simulink model "MIL4L3_SW6_V1_20220211"  (R2018b)
settings: Solver=FixedStepAuto  StartTime=0.0  StopTime=inf  FixedStep=0.001  RelTol=1e-3
PreLoadFcn:
  | A0_MILtest;
undefined symbols (not defined in the file or in its folder): Clb_ICADirect_LaneDisp_StateFive, Clb_ICADirect_LaneDisp_StateFour, Clb_ICADirect_LaneDisp_StateOne, Clb_ICADirect_LaneDisp_StateThree, Clb_ICADirect_LaneDisp_StateTwo, Clb_ICADirect_LaneDisp_StateZero, Clb_ICADirect_LaneDispSW, Clb_ICADirect_TrnLghtsCom_Switch, Clb_ICADirect_TrnLghtsCom_Value, Clb_ICADirect_TrnLghtsCrtl_Inhb, IMAP_Clb_ACU_Driver_Belt, IMAP_Clb_ACU_Driver_Belt_Over, IMAP_Clb_ACU_Passenger_Belt, IMAP_Clb_ACU_Passenger_Belt_Over, IMAP_Clb_ACU_RearLeft_Belt, IMAP_Clb_ACU_RearLeft_Belt_Over, IMAP_Clb_ACU_RearMiddle_Belt, IMAP_Clb_ACU_RearMiddle_Belt_Over, IMAP_Clb_ACU_RearRight_Belt, IMAP_Clb_ACU_RearRight_Belt_Over, IMAP_Clb_AEB_Switch, IMAP_Clb_AEB_Switch_Over, IMAP_Clb_ALC_TLC_Mode, IMAP_Clb_ALC_TLC_Mode_Over, IMAP_Clb_BCM_Battery_Voltage, IMAP_Clb_BCM_Battery_Voltage_Over, IMAP_Clb_BCM_BrakeLamp_State, IMAP_Clb_BCM_BrakeLamp_State_Over, IMAP_Clb_BCM_CHMSL_Status, IMAP_Clb_BCM_CHMSL_Status_Over, IMAP_Clb_BCM_Door_Lock_State, IMAP_Clb_BCM_Door_Lock_State_Over, IMAP_Clb_BCM_FrontWiper_State, IMAP_Clb_BCM_FrontWiper_State_Over, IMAP_Clb_BCM_FrontWiper_Switch, IMAP_Clb_BCM_FrontWiper_Switch_Over, IMAP_Clb_BCM_HazardLamp, IMAP_Clb_BCM_HazardLamp_Over, IMAP_Clb_BCM_HazardLamp_Switch, IMAP_Clb_BCM_HazardLamp_Switch_Over, IMAP_Clb_BCM_HighBeam_State, IMAP_Clb_BCM_HighBeam_State_Over, IMAP_Clb_BCM_Ignition_State, IMAP_Clb_BCM_Ignition_State_Over, IMAP_Clb_BCM_IHBC_Enabled, IMAP_Clb_BCM_IHBC_Enabled_Over, IMAP_Clb_BCM_Left_Light, IMAP_Clb_BCM_Left_Light_Over, IMAP_Clb_BCM_LeftTurn_Switch, IMAP_Clb_BCM_LeftTurn_Switch_Over, IMAP_Clb_BCM_LF_Door_State, IMAP_Clb_BCM_LF_Door_State_Over, IMAP_Clb_BCM_LowBeam_State, IMAP_Clb_BCM_LowBeam_State_Over, IMAP_Clb_BCM_LR_Door_State, IMAP_Clb_BCM_LR_Door_State_Over, IMAP_Clb_BCM_RF_Door_State, IMAP_Clb_BCM_RF_Door_State_Over, IMAP_Clb_BCM_Right_Light, IMAP_Clb_BCM_Right_Light_Over ... (+547)
libraries: CarMaker4SL x2153, simulink x292, dspstat3 x3, canmsglib x2, simulink_extras x1
(part 51 of 52)

== system MIL4L3_SW6_V1_20220211/CarMaker/VehicleControl/Function/LKA/LKAS1/LL/LLOn/LL State Determination (LLStateDet)/LL State Machine Conditions (LLSMCon)/Deactivation Condition (DeactvC)/Deviation Threshold Condition (DvtThresCon)/Deviation Threshold Judgement LKA (DvtThresJdg)/Deviation Speed Detection (DvtSpdDet)/Ph2SWA ==
  Action Port : ActionPort  InitializeStates=reset  ActionType=elseif
      settings: AttributesFormatString=states = %<InitializeStates>
  Constant : Constant  Value=-1  OutDataTypeStr=single
  Out : Outport
      settings: AttributesFormatString=%<OutputWhenDisabled> = %<InitialOutput>
  wires:
  Constant/1 -> Out/1

== system MIL4L3_SW6_V1_20220211/CarMaker/VehicleControl/Function/LKA/LKAS1/LL/LLOn/LL State Determination (LLStateDet)/LL State Machine Conditions (LLSMCon)/Deactivation Condition (DeactvC)/Deviation Threshold Condition (DvtThresCon)/Deviation Threshold Judgement LKA (DvtThresJdg)/Deviation Speed Detection (DvtSpdDet)/Ph3SWA ==
  Action Port : ActionPort  InitializeStates=reset  ActionType=else
      settings: AttributesFormatString=states = %<InitializeStates>
  Constant : Constant  Value=0  OutDataTypeStr=single
  Out : Outport
      settings: AttributesFormatString=%<OutputWhenDisabled> = %<InitialOutput>
  wires:
  Constant/1 -> Out/1

== system MIL4L3_SW6_V1_20220211/CarMaker/VehicleControl/Function/LKA/LKAS1/LL/LLOn/LL State Determination (LLStateDet)/LL State Machine Conditions (LLSMCon)/Disable Condition (DisblC)/Driver Intent Condition (DrvInttC)/Take-Over Steering Check (TkOvStChk)/Time Delay (TDel)/If Action Subsystem ==
  Action Port : ActionPort  InitializeStates=reset  ActionType=then
      settings: AttributesFormatString=states = %<InitializeStates>
  Constant : Constant  OutDataTypeStr=boolean  SampleTime=-1
  Out : Outport
      settings: AttributesFormatString=%<OutputWhenDisabled> = %<InitialOutput>
  wires:
  Constant/1 -> Out/1

== system MIL4L3_SW6_V1_20220211/CarMaker/VehicleControl/Function/LKA/LKAS1/LL/LLOn/LL State Determination (LLStateDet)/LL State Machine Conditions (LLSMCon)/Disable Condition (DisblC)/Driver Intent Condition (DrvInttC)/Take-Over Steering Check (TkOvStChk)/Time Delay (TDel)/If Action Subsystem3 ==
  In1 : Inport
  Action Port : ActionPort  InitializeStates=reset  ActionType=else
      settings: AttributesFormatString=states = %<InitializeStates>
  Out : Outport
      settings: AttributesFormatString=%<OutputWhenDisabled> = %<InitialOutput>
  wires:
  In1/1 -> Out/1

== system MIL4L3_SW6_V1_20220211/CarMaker/VehicleControl/Function/LKA/LKAS1/LL/LLOn/LL State Determination (LLStateDet)/LL State Machine Conditions (LLSMCon)/Disable Condition (DisblC)/Driver Intent Condition (DrvInttC)/Take-Over Steering Check (TkOvStChk)/Time Delay (TDel)/Sum Condition1 ==
  SampleTime : Inport
  Sum : Inport  Port=2
  state = reset : EnablePort  StatesWhenEnabling=reset
  Add1 : Sum  OutDataTypeStr=single
  Memory : Memory  InheritSampleTime=on
  Relational Operator : RelationalOperator  Operator=<=  OutDataTypeStr=boolean  RndMeth=Nearest
  Saturation : Saturate  UpperLimit=10  LowerLimit=0
      settings: AttributesFormatString="Min = %<LowerLimit>  Max = %<UpperLimit>"
  Out : Outport  OutputWhenDisabled=reset  InitialOutput=0
      settings: AttributesFormatString=%<OutputWhenDisabled> = %<InitialOutput>
  wires:
  Memory/1 -> Add1/2
  Add1/1 -> Saturation/1
  SampleTime/1 -> Add1/1
  Sum/1 -> Relational Operator/2
  Relational Operator/1 -> Out/1
  Saturation/1 -> Memory/1, Relational Operator/1

== system MIL4L3_SW6_V1_20220211/CarMaker/VehicleControl/OMAP/OMAP1/Runnable_OMAP_10ms_sys/OMAP_Module/ICA_Direct_G59/ICA_Define/Subsystem1/Dspl/DsplPrcs/Txt/TxtActv/Hold ==
  In1 : Inport
  Action Port : ActionPort  ActionType=else
  Out1 : Outport
  wires:
  In1/1 -> Out1/1

== system MIL4L3_SW6_V1_20220211/CarMaker/VehicleControl/OMAP/OMAP1/Runnable_OMAP_10ms_sys/OMAP_Module/ICA_Direct_G59/ICA_Define/Subsystem1/Dspl/DsplPrcs/Txt/TxtActv/Start ==
  In1 : Inport
  Action Port : ActionPort  ActionType=then
  Out1 : Outport
  wires:
  In1/1 -> Out1/1

== system MIL4L3_SW6_V1_20220211/CarMaker/VehicleControl/OMAP/OMAP1/Runnable_OMAP_10ms_sys/OMAP_Module/ICA_Direct_G59/ICA_Define/Subsystem1/Dspl/DsplPrcs/Txt/TxtActv/Stop ==
  In1 : Inport
  Action Port : ActionPort  ActionType=elseif
  Out1 : Outport
  wires:
  In1/1 -> Out1/1

== system MIL4L3_SW6_V1_20220211/CarMaker/VehicleControl/OMAP/OMAP1/Runnable_OMAP_10ms_sys/OMAP_Module/ICA_Direct_G59/ICA_Define/Subsystem1/Dspl/DsplPrcs/Txt/TxtCncl/Hold ==
  In1 : Inport
  Action Port : ActionPort  ActionType=else
  Out1 : Outport
  wires:
  In1/1 -> Out1/1

== system MIL4L3_SW6_V1_20220211/CarMaker/VehicleControl/OMAP/OMAP1/Runnable_OMAP_10ms_sys/OMAP_Module/ICA_Direct_G59/ICA_Define/Subsystem1/Dspl/DsplPrcs/Txt/TxtCncl/Start ==
  In1 : Inport
  Action Port : ActionPort  ActionType=then
  Out1 : Outport
  wires:
  In1/1 -> Out1/1

== system MIL4L3_SW6_V1_20220211/CarMaker/VehicleControl/OMAP/OMAP1/Runnable_OMAP_10ms_sys/OMAP_Module/ICA_Direct_G59/ICA_Define/Subsystem1/Dspl/DsplPrcs/Txt/TxtCncl/Stop ==
  In1 : Inport
  Action Port : ActionPort  ActionType=elseif
  Out1 : Outport
  wires:
  In1/1 -> Out1/1

== system MIL4L3_SW6_V1_20220211/CarMaker/VehicleControl/OMAP/OMAP1/Runnable_OMAP_10ms_sys/OMAP_Module/ICA_Direct_G59/ICA_Define/Subsystem1/Dspl/DsplPrcs/Txt/TxtDegraded/Hold ==
  In1 : Inport
  Action Port : ActionPort  ActionType=else
  Out1 : Outport
  wires:
  In1/1 -> Out1/1

== system MIL4L3_SW6_V1_20220211/CarMaker/VehicleControl/OMAP/OMAP1/Runnable_OMAP_10ms_sys/OMAP_Module/ICA_Direct_G59/ICA_Define/Subsystem1/Dspl/DsplPrcs/Txt/TxtDegraded/Start ==
  In1 : Inport
  Action Port : ActionPort  ActionType=then
  Out1 : Outport
  wires:
  In1/1 -> Out1/1

== system MIL4L3_SW6_V1_20220211/CarMaker/VehicleControl/OMAP/OMAP1/Runnable_OMAP_10ms_sys/OMAP_Module/ICA_Direct_G59/ICA_Define/Subsystem1/Dspl/DsplPrcs/Txt/TxtDegraded/Stop ==
  In1 : Inport
  Action Port : ActionPort  ActionType=elseif
  Out1 : Outport
  wires:
  In1/1 -> Out1/1

== system MIL4L3_SW6_V1_20220211/CarMaker/VehicleControl/OMAP/OMAP1/Runnable_OMAP_10ms_sys/OMAP_Module/ICA_Direct_G59/ICA_Define/Subsystem1/Dspl/DsplPrcs/Txt/TxtFromACC/Enabled Subsystem ==
  Num : Inport
  Enable : EnablePort  StatesWhenEnabling=reset
  Add : Sum
  Constant : Constant  OutDataTypeStr=single
  Constant1 : Constant  Value=0  OutDataTypeStr=single
  Delay : Delay  DelayLength=1  InitialCondition=0
  Gain : Gain  Gain=2  ParamDataTypeStr=single
  Relational Operator : RelationalOperator  Operator=<=  OutDataTypeStr=boolean  RndMeth=Nearest
  Saturation Dynamic : simulink/Discontinuities/Saturation Dynamic  OutMin=[]  OutMax=[]  OutDataTypeStr=Inherit: Same as second input  OutDataType=fixdt(1, 16)  OutScaling=2^-10  DoSatur=off
  Triger : Outport  OutputWhenDisabled=reset  InitialOutput=single(0)
  wires:
  Constant/1 -> Add/1
  Delay/1 -> Add/2
  Add/1 -> Saturation Dynamic/2
  Saturation Dynamic/1 -> Relational Operator/2, Delay/1
  Constant1/1 -> Saturation Dynamic/3
  Num/1 -> Relational Operator/1, Gain/1
  Gain/1 -> Saturation Dynamic/1
  Relational Operator/1 -> Triger/1

== system MIL4L3_SW6_V1_20220211/CarMaker/VehicleControl/OMAP/OMAP1/Runnable_OMAP_10ms_sys/OMAP_Module/ICA_Direct_G59/ICA_Define/Subsystem1/Dspl/DsplPrcs/Txt/TxtFromACC/Hold ==
  In1 : Inport
  Action Port : ActionPort  ActionType=else
  Out1 : Outport
  wires:
  In1/1 -> Out1/1

== system MIL4L3_SW6_V1_20220211/CarMaker/VehicleControl/OMAP/OMAP1/Runnable_OMAP_10ms_sys/OMAP_Module/ICA_Direct_G59/ICA_Define/Subsystem1/Dspl/DsplPrcs/Txt/TxtFromACC/RdrBlkInhib ==
  RdrBlkInhib_stTHState : Inport
  RdrBlkInhib_stLstTHState : Inport  Port=2
  RdrBlkInhib_stACCTxtDspl : Inport  Port=3
  Constant1 : Constant  OutDataTypeStr=uint16
  Constant2 : Constant  Value=0  OutDataTypeStr=uint16
  If : If  NumInputs=3  IfExpression=u1 == 5 & u2 == 0 & u3 == 2  ElseIfExpressions=u1 ~= 5 | u3 ~= 2
  Inhibit : Subsystem  TreatAsAtomicUnit=on
  Merge : Merge  Inputs=3
  Unit Delay1 : UnitDelay  SampleTime=-1
  hold_last : Subsystem  TreatAsAtomicUnit=on
  not_Inhibit : Subsystem  TreatAsAtomicUnit=on
  RdrBlkInhib_stRdrBlkInhibFlg : Outport
  wires:
  RdrBlkInhib_stTHState/1 -> If/1
  Merge/1 -> Unit Delay1/1, RdrBlkInhib_stRdrBlkInhibFlg/1
  Inhibit/1(Out1) -> Merge/1
  RdrBlkInhib_stLstTHState/1 -> If/2
  RdrBlkInhib_stACCTxtDspl/1 -> If/3
  Constant1/1 -> Inhibit/1(In1)
  If/1 -> Inhibit/Action
  Constant2/1 -> not_Inhibit/1(In1)
  If/2 -> not_Inhibit/Action
  Unit Delay1/1 -> hold_last/1(In1)
  If/3 -> hold_last/Action
  not_Inhibit/1(Out1) -> Merge/2
  hold_last/1(Out1) -> Merge/3

== system MIL4L3_SW6_V1_20220211/CarMaker/VehicleControl/OMAP/OMAP1/Runnable_OMAP_10ms_sys/OMAP_Module/ICA_Direct_G59/ICA_Define/Subsystem1/Dspl/DsplPrcs/Txt/TxtFromACC/Start ==
  In1 : Inport
  Action Port : ActionPort  ActionType=then
  Out1 : Outport
  wires:
  In1/1 -> Out1/1

== system MIL4L3_SW6_V1_20220211/CarMaker/VehicleControl/OMAP/OMAP1/Runnable_OMAP_10ms_sys/OMAP_Module/ICA_Direct_G59/ICA_Define/Subsystem1/Dspl/DsplPrcs/Txt/TxtFromACC/Start1 ==
  In1 : Inport
  Action Port : ActionPort  ActionType=then
  Out1 : Outport
  wires:
  In1/1 -> Out1/1

== system MIL4L3_SW6_V1_20220211/CarMaker/VehicleControl/OMAP/OMAP1/Runnable_OMAP_10ms_sys/OMAP_Module/ICA_Direct_G59/ICA_Define/Subsystem1/Dspl/DsplPrcs/Txt/TxtFromACC/Start2 ==
  In1 : Inport
  Action Port : ActionPort  ActionType=then
  Out1 : Outport
  wires:
  In1/1 -> Out1/1

== system MIL4L3_SW6_V1_20220211/CarMaker/VehicleControl/OMAP/OMAP1/Runnable_OMAP_10ms_sys/OMAP_Module/ICA_Direct_G59/ICA_Define/Subsystem1/Dspl/DsplPrcs/Txt/TxtFromACC/Start3 ==
  In1 : Inport
  Action Port : ActionPort  ActionType=then
  Out1 : Outport
  wires:
  In1/1 -> Out1/1

== system MIL4L3_SW6_V1_20220211/CarMaker/VehicleControl/OMAP/OMAP1/Runnable_OMAP_10ms_sys/OMAP_Module/ICA_Direct_G59/ICA_Define/Subsystem1/Dspl/DsplPrcs/Txt/TxtFromACC/Start4 ==
  In1 : Inport
  Action Port : ActionPort  ActionType=then
  Out1 : Outport
  wires:
  In1/1 -> Out1/1

== system MIL4L3_SW6_V1_20220211/CarMaker/VehicleControl/OMAP/OMAP1/Runnable_OMAP_10ms_sys/OMAP_Module/ICA_Direct_G59/ICA_Define/Subsystem1/Dspl/DsplPrcs/Txt/TxtFromACC/Start5 ==
  In1 : Inport
  Action Port : ActionPort  ActionType=then
  Out1 : Outport
  wires:
  In1/1 -> Out1/1

== system MIL4L3_SW6_V1_20220211/CarMaker/VehicleControl/OMAP/OMAP1/Runnable_OMAP_10ms_sys/OMAP_Module/ICA_Direct_G59/ICA_Define/Subsystem1/Dspl/DsplPrcs/Txt/TxtFromACC/Start6 ==
  In1 : Inport
  Action Port : ActionPort  ActionType=then
  Out1 : Outport
  wires:
  In1/1 -> Out1/1

== system MIL4L3_SW6_V1_20220211/CarMaker/VehicleControl/OMAP/OMAP1/Runnable_OMAP_10ms_sys/OMAP_Module/ICA_Direct_G59/ICA_Define/Subsystem1/Dspl/DsplPrcs/Txt/TxtFromACC/Start7 ==
  In1 : Inport
  Action Port : ActionPort  ActionType=then
  Out1 : Outport
  wires:
  In1/1 -> Out1/1

== system MIL4L3_SW6_V1_20220211/CarMaker/VehicleControl/OMAP/OMAP1/Runnable_OMAP_10ms_sys/OMAP_Module/ICA_Direct_G59/ICA_Define/Subsystem1/Dspl/DsplPrcs/Txt/TxtFromACC/Start8 ==
  In1 : Inport
  Action Port : ActionPort  ActionType=then
  Out1 : Outport
  wires:
  In1/1 -> Out1/1

== system MIL4L3_SW6_V1_20220211/CarMaker/VehicleControl/OMAP/OMAP1/Runnable_OMAP_10ms_sys/OMAP_Module/ICA_Direct_G59/ICA_Define/Subsystem1/Dspl/DsplPrcs/Txt/TxtFromACC/Start9 ==
  In1 : Inport
  Action Port : ActionPort  ActionType=then
  Out1 : Outport
  wires:
  In1/1 -> Out1/1

== system MIL4L3_SW6_V1_20220211/CarMaker/VehicleControl/OMAP/OMAP1/Runnable_OMAP_10ms_sys/OMAP_Module/ICA_Direct_G59/ICA_Define/Subsystem1/Dspl/DsplPrcs/Txt/TxtFromACC/Stop ==
  In1 : Inport
  Action Port : ActionPort  ActionType=else
  Out1 : Outport
  wires:
  In1/1 -> Out1/1

== system MIL4L3_SW6_V1_20220211/CarMaker/VehicleControl/OMAP/OMAP1/Runnable_OMAP_10ms_sys/OMAP_Module/ICA_Direct_G59/ICA_Define/Subsystem1/Dspl/DsplPrcs/Txt/TxtFromACC/Stop1 ==
  In1 : Inport
  Action Port : ActionPort  ActionType=else
  Out1 : Outport
  wires:
  In1/1 -> Out1/1

== system MIL4L3_SW6_V1_20220211/CarMaker/VehicleControl/OMAP/OMAP1/Runnable_OMAP_10ms_sys/OMAP_Module/ICA_Direct_G59/ICA_Define/Subsystem1/Dspl/DsplPrcs/Txt/TxtFromACC/Stop2 ==
  In1 : Inport
  Action Port : ActionPort  ActionType=else
  Out1 : Outport
  wires:
  In1/1 -> Out1/1

== system MIL4L3_SW6_V1_20220211/CarMaker/VehicleControl/OMAP/OMAP1/Runnable_OMAP_10ms_sys/OMAP_Module/ICA_Direct_G59/ICA_Define/Subsystem1/Dspl/DsplPrcs/Txt/TxtFromACC/Stop3 ==
  In1 : Inport
  Action Port : ActionPort  ActionType=else
  Out1 : Outport
  wires:
  In1/1 -> Out1/1

== system MIL4L3_SW6_V1_20220211/CarMaker/VehicleControl/OMAP/OMAP1/Runnable_OMAP_10ms_sys/OMAP_Module/ICA_Direct_G59/ICA_Define/Subsystem1/Dspl/DsplPrcs/Txt/TxtFromACC/Stop4 ==
  In1 : Inport
  Action Port : ActionPort  ActionType=elseif
  Out1 : Outport
  wires:
  In1/1 -> Out1/1

== system MIL4L3_SW6_V1_20220211/CarMaker/VehicleControl/OMAP/OMAP1/Runnable_OMAP_10ms_sys/OMAP_Module/ICA_Direct_G59/ICA_Define/Subsystem1/Dspl/DsplPrcs/Txt/TxtFromACC/Stop5 ==
  In1 : Inport
  Action Port : ActionPort  ActionType=else
  Out1 : Outport
  wires:
  In1/1 -> Out1/1

== system MIL4L3_SW6_V1_20220211/CarMaker/VehicleControl/OMAP/OMAP1/Runnable_OMAP_10ms_sys/OMAP_Module/ICA_Direct_G59/ICA_Define/Subsystem1/Dspl/DsplPrcs/Txt/TxtFromACC/Stop6 ==
  In1 : Inport
  Action Port : ActionPort  ActionType=else
  Out1 : Outport
  wires:
  In1/1 -> Out1/1

== system MIL4L3_SW6_V1_20220211/CarMaker/VehicleControl/OMAP/OMAP1/Runnable_OMAP_10ms_sys/OMAP_Module/ICA_Direct_G59/ICA_Define/Subsystem1/Dspl/DsplPrcs/Txt/TxtFromACC/Stop7 ==
  In1 : Inport
  Action Port : ActionPort  ActionType=else
  Out1 : Outport
  wires:
  In1/1 -> Out1/1

== system MIL4L3_SW6_V1_20220211/CarMaker/VehicleControl/OMAP/OMAP1/Runnable_OMAP_10ms_sys/OMAP_Module/ICA_Direct_G59/ICA_Define/Subsystem1/Dspl/DsplPrcs/Txt/TxtFromACC/Stop8 ==
  In1 : Inport
  Action Port : ActionPort  ActionType=else
  Out1 : Outport
  wires:
  In1/1 -> Out1/1

== system MIL4L3_SW6_V1_20220211/CarMaker/VehicleControl/OMAP/OMAP1/Runnable_OMAP_10ms_sys/OMAP_Module/ICA_Direct_G59/ICA_Define/Subsystem1/Dspl/DsplPrcs/Txt/TxtFromACC/Stop9 ==
  In1 : Inport
  Action Port : ActionPort  ActionType=else
  Out1 : Outport
  wires:
  In1/1 -> Out1/1

== system MIL4L3_SW6_V1_20220211/CarMaker/VehicleControl/OMAP/OMAP1/Runnable_OMAP_10ms_sys/OMAP_Module/ICA_Direct_G59/ICA_Define/Subsystem1/Dspl/DsplPrcs/Txt/TxtInactv/Hold ==
  In1 : Inport
  Action Port : ActionPort  ActionType=else
  Out1 : Outport
  wires:
  In1/1 -> Out1/1

== system MIL4L3_SW6_V1_20220211/CarMaker/VehicleControl/OMAP/OMAP1/Runnable_OMAP_10ms_sys/OMAP_Module/ICA_Direct_G59/ICA_Define/Subsystem1/Dspl/DsplPrcs/Txt/TxtInactv/Start ==
  In1 : Inport
  Action Port : ActionPort  ActionType=elseif
  Out1 : Outport
  wires:
  In1/1 -> Out1/1

== system MIL4L3_SW6_V1_20220211/CarMaker/VehicleControl/OMAP/OMAP1/Runnable_OMAP_10ms_sys/OMAP_Module/ICA_Direct_G59/ICA_Define/Subsystem1/Dspl/DsplPrcs/Txt/TxtInactv/Stop ==
  In1 : Inport
  Action Port : ActionPort  ActionType=then
  Out1 : Outport
  wires:
  In1/1 -> Out1/1

== system MIL4L3_SW6_V1_20220211/CarMaker/VehicleControl/OMAP/OMAP1/Runnable_OMAP_10ms_sys/OMAP_Module/ICA_Direct_G59/ICA_Define/Subsystem1/Dspl/DsplPrcs/Txt/TxtOff/Hold ==
  In1 : Inport
  Action Port : ActionPort  ActionType=else
  Out1 : Outport
  wires:
  In1/1 -> Out1/1

== system MIL4L3_SW6_V1_20220211/CarMaker/VehicleControl/OMAP/OMAP1/Runnable_OMAP_10ms_sys/OMAP_Module/ICA_Direct_G59/ICA_Define/Subsystem1/Dspl/DsplPrcs/Txt/TxtOff/Start ==
  In1 : Inport
  Action Port : ActionPort  ActionType=then
  Out1 : Outport
  wires:
  In1/1 -> Out1/1

== system MIL4L3_SW6_V1_20220211/CarMaker/VehicleControl/OMAP/OMAP1/Runnable_OMAP_10ms_sys/OMAP_Module/ICA_Direct_G59/ICA_Define/Subsystem1/Dspl/DsplPrcs/Txt/TxtOff/Stop ==
  In1 : Inport
  Action Port : ActionPort  ActionType=elseif
  Out1 : Outport
  wires:
  In1/1 -> Out1/1

== system MIL4L3_SW6_V1_20220211/CarMaker/VehicleControl/OMAP/OMAP1/Runnable_OMAP_10ms_sys/OMAP_Module/ICA_Direct_G59/ICA_Define/Subsystem1/Dspl/DsplPrcs/Txt/TxtOffToFault/Hold ==
  In1 : Inport
  Action Port : ActionPort  ActionType=else
  Out1 : Outport
  wires:
  In1/1 -> Out1/1

== system MIL4L3_SW6_V1_20220211/CarMaker/VehicleControl/OMAP/OMAP1/Runnable_OMAP_10ms_sys/OMAP_Module/ICA_Direct_G59/ICA_Define/Subsystem1/Dspl/DsplPrcs/Txt/TxtOffToFault/Start ==
  In1 : Inport
  Action Port : ActionPort  ActionType=then
  Out1 : Outport
  wires:
  In1/1 -> Out1/1

== system MIL4L3_SW6_V1_20220211/CarMaker/VehicleControl/OMAP/OMAP1/Runnable_OMAP_10ms_sys/OMAP_Module/ICA_Direct_G59/ICA_Define/Subsystem1/Dspl/DsplPrcs/Txt/TxtOffToFault/Stop ==
  In1 : Inport
  Action Port : ActionPort  ActionType=elseif
  Out1 : Outport
  wires:
  In1/1 -> Out1/1

== system MIL4L3_SW6_V1_20220211/CarMaker/VehicleControl/OMAP/OMAP1/Runnable_OMAP_10ms_sys/OMAP_Module/ICA_Direct_G59/ICA_Define/Subsystem1/Dspl/DsplPrcs/Txt/TxtOn/Hold ==
  In1 : Inport
  Action Port : ActionPort  ActionType=else
  Out1 : Outport
  wires:
  In1/1 -> Out1/1

== system MIL4L3_SW6_V1_20220211/CarMaker/VehicleControl/OMAP/OMAP1/Runnable_OMAP_10ms_sys/OMAP_Module/ICA_Direct_G59/ICA_Define/Subsystem1/Dspl/DsplPrcs/Txt/TxtOn/Start ==
  In1 : Inport
  Action Port : ActionPort  ActionType=then
  Out1 : Outport
  wires:
  In1/1 -> Out1/1

== system MIL4L3_SW6_V1_20220211/CarMaker/VehicleControl/OMAP/OMAP1/Runnable_OMAP_10ms_sys/OMAP_Module/ICA_Direct_G59/ICA_Define/Subsystem1/Dspl/DsplPrcs/Txt/TxtOn/Stop ==
  In1 : Inport
  Action Port : ActionPort  ActionType=elseif
  Out1 : Outport
  wires:
  In1/1 -> Out1/1

== system MIL4L3_SW6_V1_20220211/CarMaker/VehicleControl/OMAP/OMAP1/Runnable_OMAP_10ms_sys/OMAP_Module/ICA_Direct_G59/ICA_Define/Subsystem1/Dspl/DsplPrcs/Txt/TxtOnToFault/Hold ==
  In1 : Inport
  Action Port : ActionPort  ActionType=else
  Out1 : Outport
  wires:
  In1/1 -> Out1/1

== system MIL4L3_SW6_V1_20220211/CarMaker/VehicleControl/OMAP/OMAP1/Runnable_OMAP_10ms_sys/OMAP_Module/ICA_Direct_G59/ICA_Define/Subsystem1/Dspl/DsplPrcs/Txt/TxtOnToFault/Start ==
  In1 : Inport
  Action Port : ActionPort  ActionType=then
  Out1 : Outport
  wires:
  In1/1 -> Out1/1

== system MIL4L3_SW6_V1_20220211/CarMaker/VehicleControl/OMAP/OMAP1/Runnable_OMAP_10ms_sys/OMAP_Module/ICA_Direct_G59/ICA_Define/Subsystem1/Dspl/DsplPrcs/Txt/TxtOnToFault/Stop ==
  In1 : Inport
  Action Port : ActionPort  ActionType=elseif
  Out1 : Outport
  wires:
  In1/1 -> Out1/1

== system MIL4L3_SW6_V1_20220211/CarMaker/VehicleControl/OMAP/OMAP1/Runnable_OMAP_10ms_sys/OMAP_Module/ICA_Direct_G59/ICA_Define/Subsystem1/Dspl/DsplPrcs/Txt/Txt_Tlimit/Hold ==
  In1 : Inport
  Action Port : ActionPort  ActionType=else
  Out1 : Outport
  wires:
  In1/1 -> Out1/1

== system MIL4L3_SW6_V1_20220211/CarMaker/VehicleControl/OMAP/OMAP1/Runnable_OMAP_10ms_sys/OMAP_Module/ICA_Direct_G59/ICA_Define/Subsystem1/Dspl/DsplPrcs/Txt/Txt_Tlimit/Start ==
  In1 : Inport
  Action Port : ActionPort  ActionType=then
  Out1 : Outport
  wires:
  In1/1 -> Out1/1

== system MIL4L3_SW6_V1_20220211/CarMaker/VehicleControl/OMAP/OMAP1/Runnable_OMAP_10ms_sys/OMAP_Module/ICA_Direct_G59/ICA_Define/Subsystem1/Dspl/DsplPrcs/Txt/Txt_Tlimit/Stop ==
  In1 : Inport
  Action Port : ActionPort  ActionType=elseif
  Out1 : Outport
  wires:
  In1/1 -> Out1/1

== system MIL4L3_SW6_V1_20220211/CarMaker/VehicleControl/OMAP/OMAP1/Runnable_OMAP_10ms_sys/OMAP_Module/ICA_Direct_G59/ICA_Define/Subsystem1/Dspl/DsplPrcs/Txt/Txt_Tlimit1/Hold ==
  In1 : Inport
  Action Port : ActionPort  ActionType=else
  Out1 : Outport
  wires:
  In1/1 -> Out1/1

== system MIL4L3_SW6_V1_20220211/CarMaker/VehicleControl/OMAP/OMAP1/Runnable_OMAP_10ms_sys/OMAP_Module/ICA_Direct_G59/ICA_Define/Subsystem1/Dspl/DsplPrcs/Txt/Txt_Tlimit1/Start ==
  In1 : Inport
  Action Port : ActionPort  ActionType=then
  Out1 : Outport
  wires:
  In1/1 -> Out1/1

== system MIL4L3_SW6_V1_20220211/CarMaker/VehicleControl/OMAP/OMAP1/Runnable_OMAP_10ms_sys/OMAP_Module/ICA_Direct_G59/ICA_Define/Subsystem1/Dspl/DsplPrcs/Txt/Txt_Tlimit1/Stop ==
  In1 : Inport
  Action Port : ActionPort  ActionType=elseif
  Out1 : Outport
  wires:
  In1/1 -> Out1/1

== system MIL4L3_SW6_V1_20220211/CarMaker/VehicleControl/OMAP/OMAP1/Runnable_OMAP_10ms_sys/OMAP_Module/ICA_Direct_G59/ICA_Define/Subsystem1/Dspl/DsplPrcs/Txt/Txt_Tlimit2/Hold ==
  In1 : Inport
  Action Port : ActionPort  ActionType=else
  Out1 : Outport
  wires:
  In1/1 -> Out1/1

== system MIL4L3_SW6_V1_20220211/CarMaker/VehicleControl/OMAP/OMAP1/Runnable_OMAP_10ms_sys/OMAP_Module/ICA_Direct_G59/ICA_Define/Subsystem1/Dspl/DsplPrcs/Txt/Txt_Tlimit2/Start ==
  In1 : Inport
  Action Port : ActionPort  ActionType=then
  Out1 : Outport
  wires:
  In1/1 -> Out1/1

== system MIL4L3_SW6_V1_20220211/CarMaker/VehicleControl/OMAP/OMAP1/Runnable_OMAP_10ms_sys/OMAP_Module/ICA_Direct_G59/ICA_Define/Subsystem1/Dspl/DsplPrcs/Txt/Txt_Tlimit2/Stop ==
  In1 : Inport
  Action Port : ActionPort  ActionType=elseif
  Out1 : Outport
  wires:
  In1/1 -> Out1/1

== system MIL4L3_SW6_V1_20220211/CarMaker/VehicleControl/OMAP/OMAP1/Runnable_OMAP_10ms_sys/OMAP_Module/ICA_Direct_G59/ICA_Define/Subsystem1/Dspl/DsplPrcs/Txt/Txt_Tlimit3/Hold ==
  In1 : Inport
  Action Port : ActionPort  ActionType=else
  Out1 : Outport
  wires:
  In1/1 -> Out1/1

== system MIL4L3_SW6_V1_20220211/CarMaker/VehicleControl/OMAP/OMAP1/Runnable_OMAP_10ms_sys/OMAP_Module/ICA_Direct_G59/ICA_Define/Subsystem1/Dspl/DsplPrcs/Txt/Txt_Tlimit3/Start ==
  In1 : Inport
  Action Port : ActionPort  ActionType=then
  Out1 : Outport
  wires:
  In1/1 -> Out1/1

== system MIL4L3_SW6_V1_20220211/CarMaker/VehicleControl/OMAP/OMAP1/Runnable_OMAP_10ms_sys/OMAP_Module/ICA_Direct_G59/ICA_Define/Subsystem1/Dspl/DsplPrcs/Txt/Txt_Tlimit3/Stop ==
  In1 : Inport
  Action Port : ActionPort  ActionType=elseif
  Out1 : Outport
  wires:
  In1/1 -> Out1/1

== system MIL4L3_SW6_V1_20220211/CarMaker/VehicleControl/OMAP/OMAP1/Runnable_OMAP_10ms_sys/OMAP_Module/ICA_Direct_G59/ICA_Define/Subsystem1/Dspl/DsplPrcs/Txt/Txt_Tlimit4/Hold ==
  In1 : Inport
  Action Port : ActionPort  ActionType=else
  Out1 : Outport
  wires:
  In1/1 -> Out1/1

== system MIL4L3_SW6_V1_20220211/CarMaker/VehicleControl/OMAP/OMAP1/Runnable_OMAP_10ms_sys/OMAP_Module/ICA_Direct_G59/ICA_Define/Subsystem1/Dspl/DsplPrcs/Txt/Txt_Tlimit4/Start ==
  In1 : Inport
  Action Port : ActionPort  ActionType=then
  Out1 : Outport
  wires:
  In1/1 -> Out1/1

== system MIL4L3_SW6_V1_20220211/CarMaker/VehicleControl/OMAP/OMAP1/Runnable_OMAP_10ms_sys/OMAP_Module/ICA_Direct_G59/ICA_Define/Subsystem1/Dspl/DsplPrcs/Txt/Txt_Tlimit4/Stop ==
  In1 : Inport
  Action Port : ActionPort  ActionType=elseif
  Out1 : Outport
  wires:
  In1/1 -> Out1/1

== system MIL4L3_SW6_V1_20220211/CarMaker/VehicleControl/OMAP/OMAP1/Runnable_OMAP_10ms_sys/OMAP_Module/ICA_Direct_G59/ICA_Define/Subsystem1/Dspl/DsplPrcs/Txt/Txt_Tlimit5/Hold ==
  In1 : Inport
  Action Port : ActionPort  ActionType=else
  Out1 : Outport
  wires:
  In1/1 -> Out1/1

== system MIL4L3_SW6_V1_20220211/CarMaker/VehicleControl/OMAP/OMAP1/Runnable_OMAP_10ms_sys/OMAP_Module/ICA_Direct_G59/ICA_Define/Subsystem1/Dspl/DsplPrcs/Txt/Txt_Tlimit5/Start ==
  In1 : Inport
  Action Port : ActionPort  ActionType=then
  Out1 : Outport
  wires:
  In1/1 -> Out1/1

== system MIL4L3_SW6_V1_20220211/CarMaker/VehicleControl/OMAP/OMAP1/Runnable_OMAP_10ms_sys/OMAP_Module/ICA_Direct_G59/ICA_Define/Subsystem1/Dspl/DsplPrcs/Txt/Txt_Tlimit5/Stop ==
  In1 : Inport
  Action Port : ActionPort  ActionType=elseif
  Out1 : Outport
  wires:
  In1/1 -> Out1/1

== system MIL4L3_SW6_V1_20220211/CarMaker/VehicleControl/OMAP/OMAP1/Runnable_OMAP_10ms_sys/OMAP_Module/ICA_Direct_G59/ICA_Define/Subsystem1/Dspl/DsplPrcs/Txt/Txt_Tlimit6/Hold ==
  In1 : Inport
  Action Port : ActionPort  ActionType=else
  Out1 : Outport
  wires:
  In1/1 -> Out1/1

== system MIL4L3_SW6_V1_20220211/CarMaker/VehicleControl/OMAP/OMAP1/Runnable_OMAP_10ms_sys/OMAP_Module/ICA_Direct_G59/ICA_Define/Subsystem1/Dspl/DsplPrcs/Txt/Txt_Tlimit6/Start ==
  In1 : Inport
  Action Port : ActionPort  ActionType=then
  Out1 : Outport
  wires:
  In1/1 -> Out1/1

== system MIL4L3_SW6_V1_20220211/CarMaker/VehicleControl/OMAP/OMAP1/Runnable_OMAP_10ms_sys/OMAP_Module/ICA_Direct_G59/ICA_Define/Subsystem1/Dspl/DsplPrcs/Txt/Txt_Tlimit6/Stop ==
  In1 : Inport
  Action Port : ActionPort  ActionType=elseif
  Out1 : Outport
  wires:
  In1/1 -> Out1/1

== system MIL4L3_SW6_V1_20220211/CarMaker/VehicleControl/OMAP/OMAP1/Runnable_OMAP_10ms_sys/OMAP_Module/ICA_Direct_G59/ICA_Define/Subsystem1/Dspl/DsplPrcs/Txt/Txt_Tlimit7/Hold ==
  In1 : Inport
  Action Port : ActionPort  ActionType=else
  Out1 : Outport
  wires:
  In1/1 -> Out1/1

== system MIL4L3_SW6_V1_20220211/CarMaker/VehicleControl/OMAP/OMAP1/Runnable_OMAP_10ms_sys/OMAP_Module/ICA_Direct_G59/ICA_Define/Subsystem1/Dspl/DsplPrcs/Txt/Txt_Tlimit7/Start ==
  In1 : Inport
  Action Port : ActionPort  ActionType=then
  Out1 : Outport
  wires:
  In1/1 -> Out1/1

== system MIL4L3_SW6_V1_20220211/CarMaker/VehicleControl/OMAP/OMAP1/Runnable_OMAP_10ms_sys/OMAP_Module/ICA_Direct_G59/ICA_Define/Subsystem1/Dspl/DsplPrcs/Txt/Txt_Tlimit7/Stop ==
  In1 : Inport
  Action Port : ActionPort  ActionType=elseif
  Out1 : Outport
  wires:
  In1/1 -> Out1/1

== system MIL4L3_SW6_V1_20220211/CarMaker/VehicleControl/OMAP/OMAP1/Runnable_OMAP_10ms_sys/OMAP_Module/ICA_Direct_G59/ICA_Define/Subsystem1/Dspl/DsplPrcs/Txt/TxtFromACC/RdrBlkInhib/Inhibit ==
  In1 : Inport
  Action Port : ActionPort  ActionType=then
  Out1 : Outport
  wires:
  In1/1 -> Out1/1

== system MIL4L3_SW6_V1_20220211/CarMaker/VehicleControl/OMAP/OMAP1/Runnable_OMAP_10ms_sys/OMAP_Module/ICA_Direct_G59/ICA_Define/Subsystem1/Dspl/DsplPrcs/Txt/TxtFromACC/RdrBlkInhib/hold_last ==
  In1 : Inport
  Action Port : ActionPort  ActionType=else
  Out1 : Outport
  wires:
  In1/1 -> Out1/1

== system MIL4L3_SW6_V1_20220211/CarMaker/VehicleControl/OMAP/OMAP1/Runnable_OMAP_10ms_sys/OMAP_Module/ICA_Direct_G59/ICA_Define/Subsystem1/Dspl/DsplPrcs/Txt/TxtFromACC/RdrBlkInhib/not_Inhibit ==
  In1 : Inport
  Action Port : ActionPort  ActionType=elseif
  Out1 : Outport
  wires:
  In1/1 -> Out1/1

== matlab function MIL4L3_SW6_V1_20220211/CarMaker/VehicleControl/Function/ICA_ALC/EPS Position Control Enable Management (EPSPCEM)_KDK1/EPS_Ctr_Disable/MATLAB Function ==
  data: stEPSCtlState input; stEPSCtlCMD output
function stEPSCtlCMD = fcn(stEPSCtlState)
    stEPSCtlCMD=uint16(2);  %select
end

== matlab function MIL4L3_SW6_V1_20220211/CarMaker/VehicleControl/Data Inport/IMAP/Runnable_IMAP_10ms_sys/Runnable_IMAP_10ms_sys/IMAP_Module/MATLAB Function ==
  data: APA_FAPA_WorkSt input; IMAP_FAPA_WorkSt output
function IMAP_FAPA_WorkSt = fcn(APA_FAPA_WorkSt)
if APA_FAPA_WorkSt == uint16(2)
    IMAP_FAPA_WorkSt = uint16(1);
else
    IMAP_FAPA_WorkSt = uint16(0);
end
end

== stateflow chart MIL4L3_SW6_V1_20220211/CarMaker/VehicleControl/OMAP/OMAP1/Runnable_OMAP_10ms_sys/OMAP_Module/ACCS_Direct/ACCS_Define/ACC_State_Synthesis(ACC_SS)/If Action Subsystem2/Subsystem4/Chart ==
  state Zero
    en:
    RAPPORT=uint8(0);
  state One
    en:
    RAPPORT=uint8(1);
  (default) -> Zero
  Zero -> One : [after(2,tick)]
  One -> Zero : [[after(2,tick)]]
  data: RAPPORT output uint8

== matlab function MIL4L3_SW6_V1_20220211/CarMaker/VehicleControl/Function/ICA_ALC/EPS Position Control Enable Management (EPSPCEM)_KDK1/EPS_Ctr_Enable/MATLAB Function ==
  data: stEPSCtlState input; stEPSCtlCMD output
function stEPSCtlCMD = fcn(stEPSCtlState)
if stEPSCtlState==uint16(0) %未授权
    stEPSCtlCMD=uint16(2);  %select
elseif stEPSCtlState==uint16(2) %可使用的
    stEPSCtlCMD=uint16(3);  %授权
elseif stEPSCtlState==uint16(1) %授权的
    stEPSCtlCMD=uint16(4);  %激活
elseif stEPSCtlState==uint16(3) %激活的
    stEPSCtlCMD=uint16(4);  %激活
else
    stEPSCtlCMD=uint16(0);  %select
end

== stateflow chart MIL4L3_SW6_V1_20220211/CarMaker/VehicleControl/Function/ICA_ALC/EPS_State_Mashine/Steering Angle Cmd Synthesis State Machine (SWASynSM) ==
  state INIT
    en:EPS_Ctr_State=0;
    du:EPS_Ctr_State=0;
  state DEF
    en:EPS_Ctr_State=4;
  state EPS_OPERATIONAL
    state AVAIL
      en:EPS_Ctr_State=2;
    state AUTH
      en:EPS_Ctr_State=1;
    state ATC
      en:EPS_Ctr_State=3;
    (default) -> AVAIL
    ATC -> AVAIL : [ EPS_CMD_KDK==2]
    AUTH -> AVAIL [order 2] : [ EPS_CMD_KDK==2]
    AVAIL -> AUTH : [EPS_CMD_KDK==3]
    AUTH -> ATC [order 1] : [EPS_CMD_KDK==4]
  (default) -> INIT
  INIT -> DEF [order 1] : [EPS_Default==1]
  DEF -> INIT : [EPS_Default~=1]
  INIT -> EPS_OPERATIONAL [order 2] : [EPS_Other_Con==1 && EPS_CMD_KDK==2]
  EPS_OPERATIONAL -> INIT [order 1] : [EPS_Other_Con==0 | EPS_CMD_KDK==1 | EPS_CMD_KDK==0]
  EPS_OPERATIONAL -> DEF [order 2] : [EPS_Default==1]
  data: EPS_CMD_KDK input uint16; EPS_Other_Con input uint16; EPS_Ctr_State output uint16; EPS_Default input uint16

== stateflow chart MIL4L3_SW6_V1_20220211/CarMaker/VehicleControl/OMAP/OMAP1/Runnable_OMAP_10ms_sys/OMAP_Module/ACCS_Direct/ACCS_Define/ACC_State_Synthesis(ACC_SS)/If Action Subsystem3/Subsystem6/Chart ==
  state Zero
    en:
    RAPPORT=uint8(0);
  state One
    en:
    RAPPORT=uint8(1);
  (default) -> Zero
  Zero -> One : [after(2,tick)]
  One -> Zero : [after(2,tick)]
  data: RAPPORT output uint8

== matlab function MIL4L3_SW6_V1_20220211/CarMaker/VehicleControl/OMAP/OMAP1/Runnable_OMAP_10ms_sys/OMAP_Module/ICA_Direct_G59/ICA_Define/ICA_EPS/EPS_Ctr_Disable/MATLAB Function ==
  data: stEPSCtlState input; stEPSCtlCMD output; ControlCMDdisable input
function stEPSCtlCMD = fcn(stEPSCtlState, ControlCMDdisable)
    stEPSCtlCMD=ControlCMDdisable;  %select
end

== matlab function MIL4L3_SW6_V1_20220211/CarMaker/VehicleControl/OMAP/OMAP1/Runnable_OMAP_10ms_sys/OMAP_Module/ICA_Direct_G59/ICA_Define/ICA_EPS/EPS_Ctr_Enable/MATLAB Function ==
  data: stEPSCtlState input; stEPSCtlCMD output; EPSCMDselect input; EPSCMDauthorized input; EPSCMDactive input
function stEPSCtlCMD = fcn(stEPSCtlState, EPSCMDselect, EPSCMDauthorized, EPSCMDactive)
if stEPSCtlState==uint16(0) %unauthorized
    stEPSCtlCMD=EPSCMDselect;  %select
elseif stEPSCtlState==uint16(2) %available
    stEPSCtlCMD=EPSCMDauthorized;  %authorized
elseif stEPSCtlState==uint16(1) %authorized
    stEPSCtlCMD=EPSCMDactive;  %active
elseif stEPSCtlState==uint16(3) %active
    stEPSCtlCMD=EPSCMDactive;  %active
else
    stEPSCtlCMD=EPSCMDselect;  %select
end

== matlab function MIL4L3_SW6_V1_20220211/CarMaker/VehicleControl/OMAP/OMAP1/Runnable_OMAP_10ms_sys/OMAP_Module/ACCS_Direct/ACCS_Define/CIPV_Data ==
  data: IMAPva_d_obj_id input; IMAPva_g_obj_pos_x input; ACCSve_d_CIPV_ID input; CIPV_ID_Longitudinal_Distance output
function CIPV_ID_Longitudinal_Distance = CIPV_Data(IMAPva_d_obj_id, IMAPva_g_obj_pos_x, ACCSve_d_CIPV_ID)
%%依据CIPV_ID求出对应的纵向距离
%分类有目标和无目标
%依据CIPV_ID值求解其在IMAPva_d_obj_id的index
CIPV_ID_Longitudinal_Distance = single(200);

if ACCSve_d_CIPV_ID ~= 0
    for i = 1:40
        if IMAPva_d_obj_id(i) == ACCSve_d_CIPV_ID
            CIPV_ID_Longitudinal_Distance = IMAPva_g_obj_pos_x(i);
        end
    end
end
end

== matlab function MIL4L3_SW6_V1_20220211/CarMaker/VehicleControl/Data Inport/IMAP/Runnable_IMAP_10ms_sys/Runnable_IMAP_10ms_sys/IMAP_Module/array_transfer10 ==
  data: HazardLamp input; output output; Left_Light input; Right_Light input
function output  = signal_transfer(HazardLamp,Left_Light,Right_Light)
if HazardLamp == uint16(1)
    output = uint16(3);
elseif Left_Light == uint16(1)
    output = uint16(2);
elseif Right_Light == uint16(1)
    output = uint16(1);
else
    output = uint16(0);
end
end

== matlab function MIL4L3_SW6_V1_20220211/CarMaker/VehicleControl/Data Inport/IMAP/Runnable_IMAP_10ms_sys/Runnable_IMAP_10ms_sys/IMAP_Module/array_transfer11 ==
  data: Trunk_State input; output output; LF_Door input; RF_Door input; RR_Door input; LR_Door input
function output  = signal_transfer(Trunk_State,LF_Door,RF_Door,RR_Door,LR_Door)
if (Trunk_State == uint16(0)) && (LF_Door == uint16(0)) && (RF_Door == uint16(0)) && (RR_Door == uint16(0)) && (LR_Door == uint16(0))
    output = uint16(0);
else
    output = uint16(1);
end
end

== stateflow chart MIL4L3_SW6_V1_20220211/CarMaker/VehicleControl/Function/LKA/EPS_State_Mashine/Steering Angle Cmd Synthesis State Machine (SWASynSM) ==
  state INIT
    en:EPS_Ctr_State=0;
  state DEF
    en:EPS_Ctr_State=4;
  state EPS_OPERATIONAL
    state AVAIL
      en:EPS_Ctr_State=2;
    state AUTH
      en:EPS_Ctr_State=1;
    state ATC
      en:EPS_Ctr_State=3;
    (default) -> AVAIL
    ATC -> AVAIL [order 1] : [ LKA_State2EPS==2]
    AVAIL -> AUTH : [LKA_State2EPS==3]
    AUTH -> AVAIL [order 2] : [ LKA_State2EPS==2]
    AUTH -> ATC [order 1] : [LKA_State2EPS==4]
    ATC -> AUTH [order 2] : [LKA_State2EPS==3]
  (default) -> INIT
  INIT -> DEF [order 2] : [LKA_State2EPS==5]
  DEF -> INIT : [LKA_State2EPS~=5]
  INIT -> EPS_OPERATIONAL [order 1] : [LKA_State2EPS==2]
  EPS_OPERATIONAL -> INIT [order 1] : [ LKA_State2EPS==1 | LKA_State2EPS==0]
  EPS_OPERATIONAL -> DEF [order 2] : [LKA_State2EPS==5]
  data: LKA_State2EPS input uint8; EPS_Ctr_State output uint8

== matlab function MIL4L3_SW6_V1_20220211/CarMaker/VehicleControl/OMAP/OMAP1/Runnable_OMAP_10ms_sys/OMAP_Module/ICA_Direct_G59/ICA_Define/Subsystem1/Count1 ==
  data: count_out output
function count_out = fcn()
%#codegen
persistent count;
if isempty(count)
    count=uint16(0);
end
count=count+uint16(1);
if count>=uint16(300)
    count=uint16(0);
end
count_out = count;

== matlab function MIL4L3_SW6_V1_20220211/CarMaker/VehicleControl/OMAP/OMAP1/Runnable_OMAP_10ms_sys/OMAP_Module/ICA_Direct_G59/ICA_Define/Subsystem1/Dspl/DsplPrcs/Txt/PrioPrcs ==
  data: HndOffFlg input; GoReqFlg input; THState input; PrioPrcs_TxtDspl output; OffFlg input; TkOvFlg input; ImmdTkOvFlg input; RdrBlkFlg input; OnToFaultFlg input; OffToFaultFlg input; CnclFlg input; OnFlg input; ActvFlg input; InactvFlg input; DegradedFlg input; PressSetFlg input; ResEPBFlg input; ResBrkPedalFlg input; ISAToOnFlg input; ISAToOffFlg input
function PrioPrcs_TxtDspl  = fcn(HndOffFlg,GoReqFlg, THState,OffFlg,TkOvFlg,ImmdTkOvFlg,RdrBlkFlg,OnToFaultFlg,OffToFaultFlg,CnclFlg,OnFlg,ActvFlg,InactvFlg,DegradedFlg,PressSetFlg, ResEPBFlg, ResBrkPedalFlg, ISAToOnFlg, ISAToOffFlg)
if(ImmdTkOvFlg == uint16(1))
    PrioPrcs_TxtDspl = uint16(9);%% Please take over the car immediately %%
elseif ((THState ~= uint16(0))&&(THState ~= uint16(5))&&(HndOffFlg == 1))
    PrioPrcs_TxtDspl = uint16(8);%% Please hold the steering wheel %%
elseif (TkOvFlg == uint16(1))
    PrioPrcs_TxtDspl = uint16(7);%% Please take over the car %%
elseif (GoReqFlg == uint16(1))
    PrioPrcs_TxtDspl = uint16(6);%% ICA go request %%
elseif (OnToFaultFlg == uint16(1))
    PrioPrcs_TxtDspl = uint16(3);%% ICA Fault %%
elseif (OffToFaultFlg == uint16(1))
    PrioPrcs_TxtDspl = uint16(3);%% ICA Fault %%
elseif (RdrBlkFlg == uint16(1))
    PrioPrcs_TxtDspl = uint16(2);%% Radar Blocked %%
elseif (OffFlg == uint16(1))
    PrioPrcs_TxtDspl = uint16(11);%% ICA OFF %%
elseif (CnclFlg == uint16(1))
    PrioPrcs_TxtDspl = uint16(10);%% ICA Canceled %%    
elseif (ActvFlg == uint16(1))
    PrioPrcs_TxtDspl = uint16(5);%% ICA Active %%
elseif (ResBrkPedalFlg == uint16(1))
    PrioPrcs_TxtDspl = uint16(15);%% Release BRAKE PEDAL then active Intelligent Cruise Assist  %%
elseif (ResEPBFlg == uint16(1))
    PrioPrcs_TxtDspl = uint16(14);%% Release EPB then reactive Intelligent Cruise Assist   %%
elseif (PressSetFlg == uint16(1))
    PrioPrcs_TxtDspl = uint16(13);%% SET- key to active Intelligent Cruise Assist    %%
elseif (InactvFlg == uint16(1))
    PrioPrcs_TxtDspl = uint16(4);%% Intelligent Cruise Assist System Activation Unsatisfied %%
elseif (OnFlg == uint16(1))
    PrioPrcs_TxtDspl = uint16(1);%% Intelligent Cruise Assist System ON %%
elseif (ISAToOnFlg == uint16(1))
    PrioPrcs_TxtDspl = uint16(16);%% Temporary speed down %%
elseif (ISAToOffFlg == uint16(1))
    PrioPrcs_TxtDspl = uint16(17);%% Accelerating to target speed %%
elseif (DegradedFlg == uint16(1))
    PrioPrcs_TxtDspl = uint16(12);%% ICA degraded %%
else
    PrioPrcs_TxtDspl = uint16(0);%% No_display %%
end

== matlab function MIL4L3_SW6_V1_20220211/CarMaker/VehicleControl/OMAP/OMAP1/Runnable_OMAP_10ms_sys/OMAP_Module/ICA_Direct_G59/ICA_Define/Subsystem1/Dspl/DsplPrcs/Voc/MATLAB_Function ==
  data: Warning_duration input; Warning output; Trigger input
function Warning = fcn(Warning_duration,Trigger)
%#codegen
persistent count;
if isempty(count)
    count=uint16(0);
end
if Trigger==uint16(1)
    count=Warning_duration;
end
if count>=uint16(1)
    count=count-uint16(1);
end
if count==uint16(0)
    Warning=uint16(0);
else
    Warning=uint16(1);
end
end

== matlab function MIL4L3_SW6_V1_20220211/CarMaker/VehicleControl/OMAP/OMAP1/Runnable_OMAP_10ms_sys/OMAP_Module/ICA_Direct_G59/ICA_Define/Subsystem1/Subsystem/MATLAB Function ==
  data: TH_Mode input; LC_Scene input; TSR_Version_Only_Sign_Type output; stLCRMode input
function TSR_Version_Only_Sign_Type = fcn(TH_Mode,LC_Scene,stLCRMode)
Left_Turn=uint16(16);
Right_Turn=uint16(15);
No_Turn=uint16(0);
ZERO=uint16(0);
ONE=uint16(1);
TWO=uint16(2);
THREE=uint16(3);
if(TH_Mode~=uint16(4))
    if(stLCRMode==TWO)
        TSR_Version_Only_Sign_Type=Left_Turn;
    elseif(stLCRMode==THREE)
        TSR_Version_Only_Sign_Type=Right_Turn;   
    else
        TSR_Version_Only_Sign_Type=No_Turn;   
    end
else
    if(LC_Scene==ONE)  %Left
       TSR_Version_Only_Sign_Type=Left_Turn;
    elseif(LC_Scene==TWO)
        TSR_Version_Only_Sign_Type=Right_Turn;   
    else
        TSR_Version_Only_Sign_Type=No_Turn;  
    end
end
end

== matlab function MIL4L3_SW6_V1_20220211/CarMaker/VehicleControl/Function/LKA/LKAS1/LL/Human Machine Interface (HMI)/HMI_Popup_Status ==
  data: HMI_Popup_Status output; stDACmode input; LKA_STATE input; HandsOff input; camera_common_fault input; Front_Camera_Blocked input; stFaultCSyn input
function HMI_Popup_Status = fcn(stDACmode,LKA_STATE,HandsOff,camera_common_fault,Front_Camera_Blocked,stFaultCSyn)
if stDACmode==2&&LKA_STATE==6 %车道保持辅助故障
    HMI_Popup_Status=uint8(6);
elseif stDACmode==2&&camera_common_fault==1&&Front_Camera_Blocked~=5  %车道保持辅助暂不可用
    HMI_Popup_Status=uint8(3);
elseif (stDACmode==2||stDACmode==1)&&(Front_Camera_Blocked==5)   %摄像头被遮挡
    HMI_Popup_Status=uint8(4);
elseif (stDACmode==2||stDACmode==1)&&HandsOff==1  %手握方向盘
    HMI_Popup_Status=uint8(2);    
elseif stDACmode==2&&(LKA_STATE==2)
    HMI_Popup_Status=uint8(1);
elseif stDACmode~=2&&stFaultCSyn==0
    HMI_Popup_Status=uint8(8);
elseif stFaultCSyn==0
    HMI_Popup_Status=uint8(7);
elseif stDACmode==2&&(LKA_STATE==0||LKA_STATE==1)
    HMI_Popup_Status=uint8(0);
else
    HMI_Popup_Status=uint8(0);
end

== stateflow chart MIL4L3_SW6_V1_20220211/CarMaker/VehicleControl/OMAP/OMAP1/Runnable_OMAP_10ms_sys/OMAP_Module/ACCS_Direct/ACCS_Define/Human_Machine_Interface(ACC_HMI)/Subsystem/Chart ==
  state ObjOutRange
    en:
    Value = uint8(5);
  state ObjInRange
    state Middle
      en:
      Value = uint8(2);
    state Far
      en:
      Value = uint8(4);
    state Close
      en:
      Value = uint8(1);
    (default) -> (junction 14)
    (junction 14) -> Far [order 2] : [Distance>single(80)]
    (junction 14) -> Close [order 1] : [Distance<=single(30)]
    (junction 14) -> Middle [order 3]
    Far -> Middle [order 1] : [(Distance>single(30))&&(Distance<single(77))]
    Middle -> Close [order 1] : [Distance<single(27)]
    Middle -> Far [order 2] : [Distance>single(80)]
    Close -> Middle [order 1] : [(Distance>single(30))&&(Distance<=single(80))]
    Close -> Far [order 2] : [Distance>single(80)]
    Far -> Close [order 2] : [Distance<=single(30)]
  (default) -> (junction 28)
  (junction 28) -> ObjInRange [order 1] : [(Distance>=single(0))&&(Distance<=single(150))]
  (junction 28) -> ObjOutRange [order 2]
  ObjInRange -> ObjOutRange : [(Distance<single(0))||(Distance>single(150))]
  ObjOutRange -> ObjInRange : [(Distance>=single(0))&&(Distance<=single(150))]
  data: Distance input; Value output uint8

== stateflow chart MIL4L3_SW6_V1_20220211/CarMaker/VehicleControl/OMAP/OMAP1/Runnable_OMAP_10ms_sys/OMAP_Module/ACCS_Direct/ACCS_Define/Human_Machine_Interface(ACC_HMI)/Text_PopUp/ Radar_Blocked/Chart ==
  state StandBy
    en:
    Value = data;
  state Trigger
    en:
    Value = data;
  (default) -> StandBy
  StandBy -> Trigger : [data==1]
  Trigger -> StandBy : [after(3,sec)]
  data: data input; Value output boolean

== stateflow chart MIL4L3_SW6_V1_20220211/CarMaker/VehicleControl/OMAP/OMAP1/Runnable_OMAP_10ms_sys/OMAP_Module/ACCS_Direct/ACCS_Define/Human_Machine_Interface(ACC_HMI)/Text_PopUp/ACC_Activation_Unsatisfied/Chart ==
  state StandBy
    en:
    Value = data;
  state Trigger
    en:
    Value = data;
  (default) -> StandBy
  StandBy -> Trigger : [data==1]
  Trigger -> StandBy : [after(3,sec)]
  data: data input; Value output boolean

== stateflow chart MIL4L3_SW6_V1_20220211/CarMaker/VehicleControl/OMAP/OMAP1/Runnable_OMAP_10ms_sys/OMAP_Module/ACCS_Direct/ACCS_Define/Human_Machine_Interface(ACC_HMI)/Text_PopUp/ACC_Active/Chart ==
  state StandBy
    en:
    Value = data;
  state Trigger
    en:
    Value = data;
  (default) -> StandBy
  StandBy -> Trigger : [data==1]
  Trigger -> StandBy : [after(3,sec)]
  data: data input; Value output boolean

== matlab function MIL4L3_SW6_V1_20220211/CarMaker/VehicleControl/Function/LKA/LKAS1/LL/Human Machine Interface (HMI)/Hands_Off_Warning ==
  data: Hands_Off_Warning output; HandsOff input
function Hands_Off_Warning = fcn(HandsOff)
if HandsOff==0
    Hands_Off_Warning= uint8(0);
elseif HandsOff==1
    Hands_Off_Warning= uint8(1);
else
    Hands_Off_Warning= uint8(0);
end

== stateflow chart MIL4L3_SW6_V1_20220211/CarMaker/VehicleControl/OMAP/OMAP1/Runnable_OMAP_10ms_sys/OMAP_Module/ACCS_Direct/ACCS_Define/Human_Machine_Interface(ACC_HMI)/Text_PopUp/ACC_Canceled/Chart ==
  state StandBy
    en:
    Value = data;
  state Trigger
    en:
    Value = data;
  (default) -> StandBy
  StandBy -> Trigger : [data==1]
  Trigger -> StandBy : [after(3,sec)]
  data: data input; Value output boolean

== stateflow chart MIL4L3_SW6_V1_20220211/CarMaker/VehicleControl/OMAP/OMAP1/Runnable_OMAP_10ms_sys/OMAP_Module/ACCS_Direct/ACCS_Define/Human_Machine_Interface(ACC_HMI)/Text_PopUp/ACC_Fault/Chart ==
  state StandBy
    en:
    Value = data;
  state Trigger
    en:
    Value = data;
  (default) -> StandBy
  StandBy -> Trigger : [data==1]
  Trigger -> StandBy : [after(3,sec)]
  data: data input; Value output boolean

== stateflow chart MIL4L3_SW6_V1_20220211/CarMaker/VehicleControl/OMAP/OMAP1/Runnable_OMAP_10ms_sys/OMAP_Module/ACCS_Direct/ACCS_Define/Human_Machine_Interface(ACC_HMI)/Text_PopUp/ACC_OFF/Chart ==
  state StandBy
    en:
    Value = data;
  state Trigger
    en:
    Value = data;
  (default) -> StandBy
  StandBy -> Trigger : [(data==1)&&(data1==0)]
  Trigger -> StandBy : [after(3,sec)]
  data: data input; Value output boolean; data1 input

== stateflow chart MIL4L3_SW6_V1_20220211/CarMaker/VehicleControl/OMAP/OMAP1/Runnable_OMAP_10ms_sys/OMAP_Module/ACCS_Direct/ACCS_Define/Human_Machine_Interface(ACC_HMI)/Text_PopUp/ACC_ON/Chart ==
  state StandBy
    en:
    Value = data;
  state Trigger
    en:
    Value = data;
  state Trigger1
    en:
    Value = data2;
  (default) -> StandBy
  StandBy -> Trigger [order 1] : [data==1]
  Trigger -> StandBy : [after(6,sec)||(data1==1)]
  Trigger1 -> StandBy : [after(6,sec)||(data1==1)]
  StandBy -> Trigger1 [order 2] : [data2==1]
  data: data input; Value output boolean; data1 input; data2 input

== stateflow chart MIL4L3_SW6_V1_20220211/CarMaker/VehicleControl/OMAP/OMAP1/Runnable_OMAP_10ms_sys/OMAP_Module/ACCS_Direct/ACCS_Define/Human_Machine_Interface(ACC_HMI)/Text_PopUp/Please_Take_Over_the_Car/Chart1 ==
  state StandBy
    en:
    Value = uint8(0);
  state Trigger
    en:
    Value = uint8(1);
  (default) -> StandBy
  StandBy -> Trigger : [IN==1]
  Trigger -> StandBy : [OUT==1]
  data: IN input boolean; OUT input boolean; Value output uint8

== stateflow chart MIL4L3_SW6_V1_20220211/CarMaker/VehicleControl/OMAP/OMAP1/Runnable_OMAP_10ms_sys/OMAP_Module/ACCS_Direct/ACCS_Define/Human_Machine_Interface(ACC_HMI)/Text_PopUp/Please_Take_Over_the_Car_immediataly/Chart1 ==
  state StandBy1
    en:
    Value = uint8(0);
  state Trigger
    en:
    Value = uint8(1);
  state StandBy
    en:
    Value = uint8(0);
  (default) -> StandBy
  StandBy -> StandBy1 : [(ESC_DecTar>-5)&&(ESC_DecTar<-3)]
  StandBy1 -> Trigger [order 2] : [after(4,sec)]
  StandBy1 -> StandBy [order 1] : [ESC_DecTar>-3]
  Trigger -> StandBy : [ESC_DecTar>-3]
  data: ESC_DecTar input single; Value output uint8; BRAKE_RELEASED_FAILSAFE input

== matlab function MIL4L3_SW6_V1_20220211/CarMaker/VehicleControl/Function/LKA/LKAS1/LL/Human Machine Interface (HMI)/LDW_Flag ==
  data: HMI_stDACmode input; HMI_LKA_STATE input; LDW_Flag output; HMI_LDWWarnInfo input
function LDW_Flag = fcn(HMI_stDACmode, HMI_LKA_STATE, HMI_LDWWarnInfo)
if HMI_stDACmode==1
    if HMI_LDWWarnInfo==1
        LDW_Flag=uint8(1);
    elseif HMI_LDWWarnInfo==2
        LDW_Flag=uint8(2);
    else
        LDW_Flag=uint8(0);
    end
elseif HMI_stDACmode==2
    if HMI_LDWWarnInfo==1 && HMI_LKA_STATE==4
        LDW_Flag=uint8(1);
    elseif HMI_LDWWarnInfo==2 && HMI_LKA_STATE==5
        LDW_Flag=uint8(2);
    else
        LDW_Flag=uint8(0);
    end    
else
    LDW_Flag=uint8(0);
end
end

== matlab function MIL4L3_SW6_V1_20220211/CarMaker/VehicleControl/Function/LKA/LKAS1/LL/Human Machine Interface (HMI)/LDW_Status_Display ==
  data: stDACmode input; LDW_Status_Display output; LDW_STATE input
function LDW_Status_Display = fcn(stDACmode,LDW_STATE)
if (stDACmode==1)&&LDW_STATE~=6
    LDW_Status_Display=uint8(1);
elseif (stDACmode==1)&&LDW_STATE==6
    LDW_Status_Display=uint8(2);
else
    LDW_Status_Display=uint8(0);
end

== matlab function MIL4L3_SW6_V1_20220211/CarMaker/VehicleControl/Function/LKA/LKAS1/LL/Human Machine Interface (HMI)/LKA_Status_Display ==
  data: stDACmode input; LKA_Status_Display output; LKA_STATE input
function LKA_Status_Display  = fcn(stDACmode,LKA_STATE)

if stDACmode==2&&LKA_STATE~=6
    LKA_Status_Display=single(1);
elseif stDACmode==2&&LKA_STATE==6
    LKA_Status_Display=single(2);
else
    LKA_Status_Display=single(0);
end

== matlab function MIL4L3_SW6_V1_20220211/CarMaker/VehicleControl/Function/LKA/LKAS1/LL/Human Machine Interface (HMI)/LKA_action_indication ==
  data: LKA_Action_Indication output; stDACmode input; LKA_STATE input
function LKA_Action_Indication = fcn(stDACmode,LKA_STATE)
if stDACmode==2&&LKA_STATE==2
    LKA_Action_Indication=uint8(1);
elseif stDACmode==2&&LKA_STATE==3
    LKA_Action_Indication=uint8(2);
elseif stDACmode==2&&(LKA_STATE==4||LKA_STATE==5)
    LKA_Action_Indication=uint8(3);
else
    LKA_Action_Indication=uint8(0);
end
